simulink library "GESHandler"  (R2016b)
settings: Solver=VariableStepAuto  StartTime=0.0  StopTime=10.0  RelTol=1e-3
undefined symbols (not defined in the file or in its folder): GES, GESError
libraries: VariousLibrary x10, TimestampChecker x3
settings Model: Creator=Nathan  LastModifiedBy=march

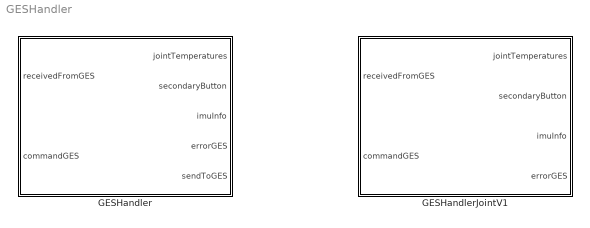
== system GESHandler ==
  GESHandler : Subsystem
  GESHandlerJointV1 : Subsystem  AncestorBlock=GESHandler/GESHandler

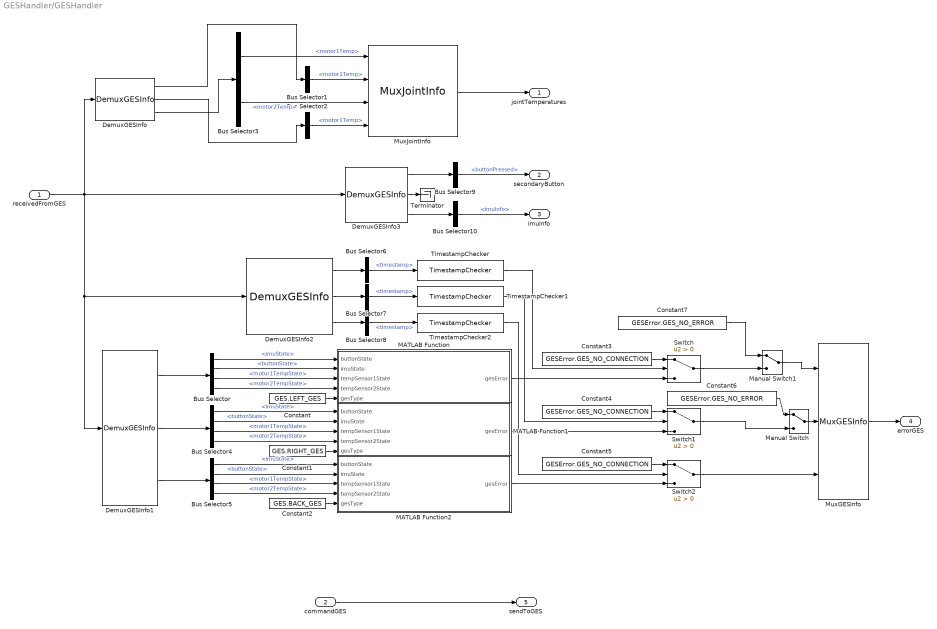
== system GESHandler/GESHandler ==
  receivedFromGES : Inport  OutDataTypeStr=Bus: EtherCATReceivedFromGES  BusOutputAsStruct=on
  commandGES : Inport  Port=2  OutDataTypeStr=Bus: GESCommand
  Bus Selector : BusSelector  OutputSignals=imuState,buttonState,motor1TempState,motor2TempState
  Bus Selector1 : BusSelector  OutputSignals=motor1Temp
  Bus Selector10 : BusSelector  OutputSignals=imuInfo
  Bus Selector2 : BusSelector  OutputSignals=motor1Temp
  Bus Selector3 : BusSelector  OutputSignals=motor1Temp,motor2Temp
  Bus Selector4 : BusSelector  OutputSignals=imuState,buttonState,motor1TempState,motor2TempState
  Bus Selector5 : BusSelector  OutputSignals=imuState,buttonState,motor1TempState,motor2TempState
  Bus Selector6 : BusSelector  OutputSignals=timestamp
  Bus Selector7 : BusSelector  OutputSignals=timestamp
  Bus Selector8 : BusSelector  OutputSignals=timestamp
  Bus Selector9 : BusSelector  OutputSignals=buttonPressed
  Constant : Constant  Value=GES.LEFT_GES
  Constant1 : Constant  Value=GES.RIGHT_GES
  Constant2 : Constant  Value=GES.BACK_GES
  Constant3 : Constant  Value=GESError.GES_NO_CONNECTION
  Constant4 : Constant  Value=GESError.GES_NO_CONNECTION
  Constant5 : Constant  Value=GESError.GES_NO_CONNECTION
  Constant6 : Constant  Value=GESError.GES_NO_ERROR
  Constant7 : Constant  Value=GESError.GES_NO_ERROR
  DemuxGESInfo{,1..3} (4 alike) : VariousLibrary/DemuxGESInfo
  MATLAB Function : MATLAB Function  TreatAsAtomicUnit=on
  MATLAB Function1 : MATLAB Function  TreatAsAtomicUnit=on
  MATLAB Function2 : MATLAB Function  TreatAsAtomicUnit=on
  Manual Switch : ManualSwitch
  Manual Switch1 : ManualSwitch
  MuxGESInfo : VariousLibrary/MuxGESInfo
  MuxJointInfo : VariousLibrary/MuxJointInfo
  Switch : Switch  Criteria=u2 > Threshold
  Switch1 : Switch  Criteria=u2 > Threshold
  Switch2 : Switch  Criteria=u2 > Threshold
  Terminator : Terminator
  TimestampChecker : TimestampChecker/TimestampChecker
  TimestampChecker1 : TimestampChecker/TimestampChecker
  TimestampChecker2 : TimestampChecker/TimestampChecker
  jointTemperatures : Outport
  secondaryButton : Outport  Port=2
  imuInfo : Outport  Port=3
  errorGES : Outport  Port=4  OutDataTypeStr=Enum: GESError  PortDimensions=[1 3]
  sendToGES : Outport  Port=5  OutDataTypeStr=Bus: GESCommand  PortDimensions=[1 3]
  wires:
  Bus Selector2/1 -> MuxJointInfo/4  "<motor1Temp>"
  Bus Selector1/1 -> MuxJointInfo/2  "<motor1Temp>"
  Bus Selector3/2 -> MuxJointInfo/3  "<motor2Temp>"
  Bus Selector3/1 -> MuxJointInfo/1  "<motor1Temp>"
  DemuxGESInfo/2 -> Bus Selector2/1
  DemuxGESInfo/3 -> Bus Selector3/1
  DemuxGESInfo/1 -> Bus Selector1/1
  receivedFromGES/1 -> DemuxGESInfo1/1, DemuxGESInfo2/1, DemuxGESInfo3/1, DemuxGESInfo/1
  MuxJointInfo/1 -> jointTemperatures/1
  MuxGESInfo/1 -> errorGES/1
  DemuxGESInfo1/1 -> Bus Selector/1
  DemuxGESInfo1/2 -> Bus Selector4/1
  DemuxGESInfo1/3 -> Bus Selector5/1
  Constant/1 -> MATLAB Function/5(gesType)
  Bus Selector/3 -> MATLAB Function/3(tempSensor1State)  "<motor1TempState>"
  Bus Selector/4 -> MATLAB Function/4(tempSensor2State)  "<motor2TempState>"
  Bus Selector/2 -> MATLAB Function/2(imuState)  "<buttonState>"
  Bus Selector/1 -> MATLAB Function/1(buttonState)  "<imuState>"
  Bus Selector4/1 -> MATLAB Function1/1(buttonState)  "<imuState>"
  Bus Selector4/4 -> MATLAB Function1/4(tempSensor2State)  "<motor2TempState>"
  Bus Selector4/3 -> MATLAB Function1/3(tempSensor1State)  "<motor1TempState>"
  Bus Selector4/2 -> MATLAB Function1/2(imuState)  "<buttonState>"
  Constant1/1 -> MATLAB Function1/5(gesType)
  Bus Selector5/3 -> MATLAB Function2/3(tempSensor1State)  "<motor1TempState>"
  Bus Selector5/4 -> MATLAB Function2/4(tempSensor2State)  "<motor2TempState>"
  Bus Selector5/1 -> MATLAB Function2/1(buttonState)  "<imuState>"
  Bus Selector5/2 -> MATLAB Function2/2(imuState)  "<buttonState>"
  Constant2/1 -> MATLAB Function2/5(gesType)
  DemuxGESInfo2/1 -> Bus Selector6/1
  DemuxGESInfo2/3 -> Bus Selector8/1
  DemuxGESInfo2/2 -> Bus Selector7/1
  Bus Selector6/1 -> TimestampChecker/1  "<timestamp>"
  Bus Selector8/1 -> TimestampChecker2/1  "<timestamp>"
  Bus Selector7/1 -> TimestampChecker1/1  "<timestamp>"
  Switch1/1 -> Manual Switch/2
  Switch/1 -> Manual Switch1/2
  Switch2/1 -> MuxGESInfo/3
  DemuxGESInfo3/1 -> Bus Selector9/1
  DemuxGESInfo3/3 -> Bus Selector10/1
  DemuxGESInfo3/2 -> Terminator/1
  Bus Selector9/1 -> secondaryButton/1  "<buttonPressed>"
  Bus Selector10/1 -> imuInfo/1  "<imuInfo>"
  Constant3/1 -> Switch/1
  Constant4/1 -> Switch1/1
  Constant5/1 -> Switch2/1
  MATLAB Function/1(gesError) -> Switch/3
  MATLAB Function1/1(gesError) -> Switch1/3
  MATLAB Function2/1(gesError) -> Switch2/3
  TimestampChecker2/1 -> Switch2/2
  TimestampChecker1/1 -> Switch1/2
  TimestampChecker/1 -> Switch/2
  commandGES/1 -> sendToGES/1
  Manual Switch1/1 -> MuxGESInfo/1
  Constant7/1 -> Manual Switch1/1
  Manual Switch/1 -> MuxGESInfo/2
  Constant6/1 -> Manual Switch/1

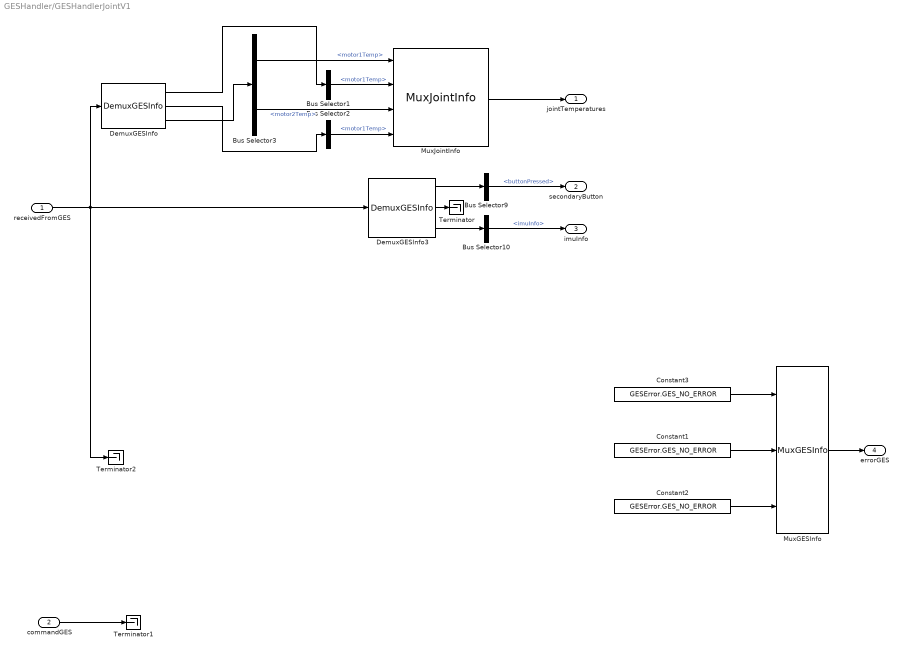
== system GESHandler/GESHandlerJointV1 ==
  receivedFromGES : Inport  OutDataTypeStr=Bus: EtherCATReceivedFromGES  BusOutputAsStruct=on
  commandGES : Inport  Port=2
  Bus Selector1 : BusSelector  OutputSignals=motor1Temp
  Bus Selector10 : BusSelector  OutputSignals=imuInfo
  Bus Selector2 : BusSelector  OutputSignals=motor1Temp
  Bus Selector3 : BusSelector  OutputSignals=motor1Temp,motor2Temp
  Bus Selector9 : BusSelector  OutputSignals=buttonPressed
  Constant1 : Constant  Value=GESError.GES_NO_ERROR
  Constant2 : Constant  Value=GESError.GES_NO_ERROR
  Constant3 : Constant  Value=GESError.GES_NO_ERROR
  DemuxGESInfo : VariousLibrary/DemuxGESInfo
  DemuxGESInfo3 : VariousLibrary/DemuxGESInfo
  MuxGESInfo : VariousLibrary/MuxGESInfo
  MuxJointInfo : VariousLibrary/MuxJointInfo
  Terminator : Terminator
  Terminator1 : Terminator
  Terminator2 : Terminator
  jointTemperatures : Outport
  secondaryButton : Outport  Port=2
  imuInfo : Outport  Port=3
  errorGES : Outport  Port=4  OutDataTypeStr=Enum: GESError  PortDimensions=[1 3]
  wires:
  commandGES/1 -> Terminator1/1
  Bus Selector10/1 -> imuInfo/1  "<imuInfo>"
  Bus Selector9/1 -> secondaryButton/1  "<buttonPressed>"
  DemuxGESInfo3/2 -> Terminator/1
  DemuxGESInfo3/3 -> Bus Selector10/1
  DemuxGESInfo3/1 -> Bus Selector9/1
  Constant2/1 -> MuxGESInfo/3
  Constant3/1 -> MuxGESInfo/1
  Constant1/1 -> MuxGESInfo/2
  MuxGESInfo/1 -> errorGES/1
  MuxJointInfo/1 -> jointTemperatures/1
  receivedFromGES/1 -> Terminator2/1, DemuxGESInfo/1, DemuxGESInfo3/1
  DemuxGESInfo/1 -> Bus Selector1/1
  DemuxGESInfo/3 -> Bus Selector3/1
  DemuxGESInfo/2 -> Bus Selector2/1
  Bus Selector3/1 -> MuxJointInfo/1  "<motor1Temp>"
  Bus Selector3/2 -> MuxJointInfo/3  "<motor2Temp>"
  Bus Selector1/1 -> MuxJointInfo/2  "<motor1Temp>"
  Bus Selector2/1 -> MuxJointInfo/4  "<motor1Temp>"

== matlab function GESHandler/MATLAB Function ==
  data: buttonState input; gesError output; imuState input; tempSensor1State input; tempSensor2State input; gesType input
function gesError   = getErrorFromGES(buttonState, imuState, tempSensor1State, tempSensor2State, gesType)
% wrapper function for getErrorFromGES;
gesError = getErrorFromGES(buttonState, imuState, tempSensor1State, tempSensor2State, gesType);
end

== matlab function GESHandler/MATLAB Function1 ==
  data: buttonState input; gesError output; imuState input; tempSensor1State input; tempSensor2State input; gesType input
function gesError   = getErrorFromGES(buttonState, imuState, tempSensor1State, tempSensor2State, gesType)
% wrapper function for getErrorFromGES;
gesError = getErrorFromGES(buttonState, imuState, tempSensor1State, tempSensor2State, gesType);
end

== matlab function GESHandler/MATLAB Function2 ==
  data: buttonState input; gesError output; imuState input; tempSensor1State input; tempSensor2State input; gesType input
function gesError   = getErrorFromGES(buttonState, imuState, tempSensor1State, tempSensor2State, gesType)
% wrapper function for getErrorFromGES;
gesError = getErrorFromGES(buttonState, imuState, tempSensor1State, tempSensor2State, gesType);
end
